simulink model "sim_quadrotor_linear_16b"  (R2016b)
settings: Solver=ode4  StartTime=0.0  StopTime=25  FixedStep=0.0001  RelTol=1e-3
values from neighbouring files (symbols this model uses):
  Par_mdlQuad = mdl_quadrotor_par()    [sim_quadrotor_linear_init.m]
undefined symbols (not defined in the file or in its folder): Ag_phi_rad, Ag_theta_rad, AgVel_p_radPerScnd, AgVel_q_radPerScnd, Pos_z_mtr, V_u_mtrPerScnd, V_v_mtrPerScnd, V_w_mtrPerScnd
settings Model: Creator=Nu  LastModifiedBy=Nu

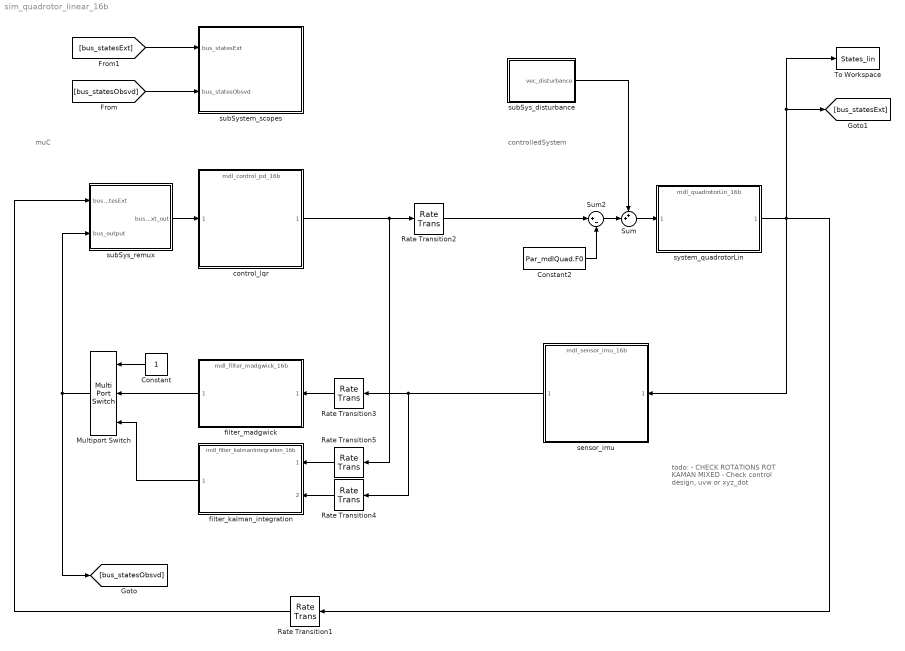
== system sim_quadrotor_linear_16b ==
  note: todo:
      | - CHECK ROTATIONS ROT KAMAN MIXED
      | - Check control design, uvw or xyz_dot
  note: controlledSystem
  note: muC
  Constant : Constant
  Constant2 : Constant  Value=Par_mdlQuad.F0
  Multiport Switch : MultiPortSwitch  DataPortOrder=Zero-based contiguous  Inputs=2
  Rate Transition1 : RateTransition
  Rate Transition2 : RateTransition
  Rate Transition3 : RateTransition  OutPortSampleTime=Par_filterMadgwick.T
  Rate Transition4 : RateTransition  OutPortSampleTime=Par_filterKalman.T
  Rate Transition5 : RateTransition  X0=Par_mdlQuad.PWM0*ones(4,1)
  Sum : Sum  Inputs=++|
  Sum2 : Sum  Inputs=|+-
  To Workspace : ToWorkspace  VariableName=States_lin  SaveFormat=Timeseries  SampleTime=-1
  control_lqr : ModelReference  ModelNameDialog=mdl_control_pd_16b.slx  SimulationMode=Normal  ModelReferenceVersion=1.259
  filter_kalman_integration : ModelReference  ModelNameDialog=mdl_filter_kalmanIntegration_16b.slx  SimulationMode=Normal  ModelReferenceVersion=1.142
  filter_madgwick : ModelReference  ModelNameDialog=mdl_filter_madgwick_16b.slx  SimulationMode=Normal  ModelReferenceVersion=1.85
  sensor_imu : ModelReference  ModelNameDialog=mdl_sensor_imu_16b.slx  SimulationMode=Normal  ModelReferenceVersion=1.279
  subSys_disturbance : Subsystem
  subSys_remux : Subsystem
  subSystem_scopes : Subsystem
  system_quadrotorLin : ModelReference  ModelNameDialog=mdl_quadrotorLin_16b.slx  SimulationMode=Normal  ModelReferenceVersion=1.303
  wires:
  system_quadrotorLin/1 -> To Workspace/1, [bus_statesExt], Rate Transition1/1, sensor_imu/1
  sensor_imu/1 -> Rate Transition4/1, Rate Transition3/1
  [bus_statesObsvd] -> subSystem_scopes/2(bus_statesObsvd)
  [bus_statesExt] -> subSystem_scopes/1(bus_statesExt)
  Multiport Switch/1 -> [bus_statesObsvd], subSys_remux/2(bus_output)
  Rate Transition3/1 -> filter_madgwick/1
  filter_kalman_integration/1 -> Multiport Switch/3
  filter_madgwick/1 -> Multiport Switch/2
  Constant/1 -> Multiport Switch/1
  Rate Transition4/1 -> filter_kalman_integration/2
  Rate Transition1/1 -> subSys_remux/1(bus_statesExt)
  subSys_remux/1(bus_statesExt_out) -> control_lqr/1
  Rate Transition5/1 -> filter_kalman_integration/1
  control_lqr/1 -> Rate Transition2/1, Rate Transition5/1
  subSys_disturbance/1(vec_disturbance) -> Sum/1
  Rate Transition2/1 -> Sum2/1
  Constant2/1 -> Sum2/2
  Sum2/1 -> Sum/2
  Sum/1 -> system_quadrotorLin/1

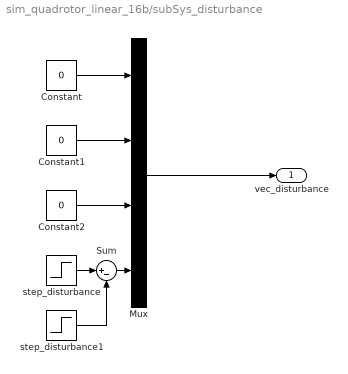
== system sim_quadrotor_linear_16b/subSys_disturbance ==
  Constant : Constant  Value=0
  Constant1 : Constant  Value=0
  Constant2 : Constant  Value=0
  Mux : Mux
  Sum : Sum  Inputs=|+-
  step_disturbance : Step  Time=10  After=0.1  SampleTime=0
  step_disturbance1 : Step  Time=10.5  After=0.1  SampleTime=0
  vec_disturbance : Outport
  wires:
  Sum/1 -> Mux/4
  Constant/1 -> Mux/1
  Constant1/1 -> Mux/2
  Constant2/1 -> Mux/3
  step_disturbance1/1 -> Sum/2
  step_disturbance/1 -> Sum/1
  Mux/1 -> vec_disturbance/1

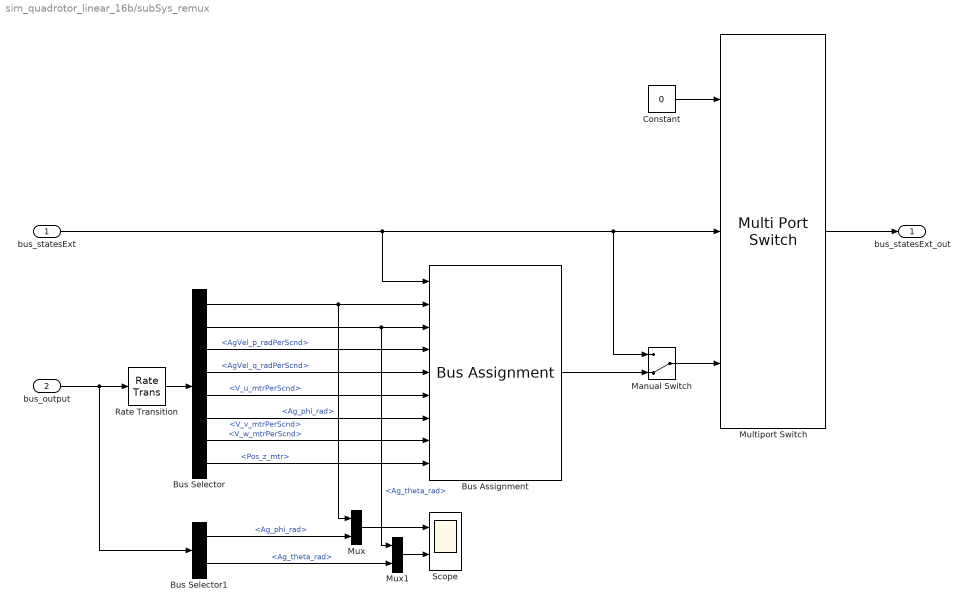
== system sim_quadrotor_linear_16b/subSys_remux ==
  bus_statesExt : Inport
  bus_output : Inport  Port=2
  Bus Assignment : BusAssignment  AssignedSignals=Ag_phi_rad,Ag_theta_rad,AgVel_p_radPerScnd,AgVel_q_radPerScnd,V_u_mtrPerScnd,V_v_mtrPerScnd,V_w_mtrPerScnd,Pos_z_mtr
  Bus Selector : BusSelector  OutputSignals=Ag_phi_rad,Ag_theta_rad,AgVel_p_radPerScnd,AgVel_q_radPerScnd,V_u_mtrPerScnd,V_v_mtrPerScnd,V_w_mtrPerScnd,Pos_z_mtr
  Bus Selector1 : BusSelector  OutputSignals=Ag_phi_rad,Ag_theta_rad
  Constant : Constant  Value=0
  Manual Switch : ManualSwitch  CurrentSetting=0
  Multiport Switch : MultiPortSwitch  DataPortOrder=Zero-based contiguous  Inputs=2
  Mux : Mux  Inputs=2
  Mux1 : Mux  Inputs=2
  Rate Transition : RateTransition
  Scope : Scope  NumInputPorts=2
  bus_statesExt_out : Outport
  wires:
  Bus Selector/2 -> Mux1/1, Bus Assignment/3  "<Ag_theta_rad>"
  Bus Selector/1 -> Mux/1, Bus Assignment/2  "<Ag_phi_rad>"
  Multiport Switch/1 -> bus_statesExt_out/1
  Constant/1 -> Multiport Switch/1
  bus_statesExt/1 -> Manual Switch/1, Multiport Switch/2, Bus Assignment/1
  bus_output/1 -> Rate Transition/1, Bus Selector1/1
  Bus Assignment/1 -> Manual Switch/2
  Rate Transition/1 -> Bus Selector/1
  Bus Selector1/1 -> Mux/2  "<Ag_phi_rad>"
  Mux/1 -> Scope/1
  Mux1/1 -> Scope/2
  Bus Selector1/2 -> Mux1/2  "<Ag_theta_rad>"
  Bus Selector/3 -> Bus Assignment/4  "<AgVel_p_radPerScnd>"
  Bus Selector/4 -> Bus Assignment/5  "<AgVel_q_radPerScnd>"
  Bus Selector/5 -> Bus Assignment/6  "<V_u_mtrPerScnd>"
  Bus Selector/6 -> Bus Assignment/7  "<V_v_mtrPerScnd>"
  Manual Switch/1 -> Multiport Switch/3
  Bus Selector/7 -> Bus Assignment/8  "<V_w_mtrPerScnd>"
  Bus Selector/8 -> Bus Assignment/9  "<Pos_z_mtr>"

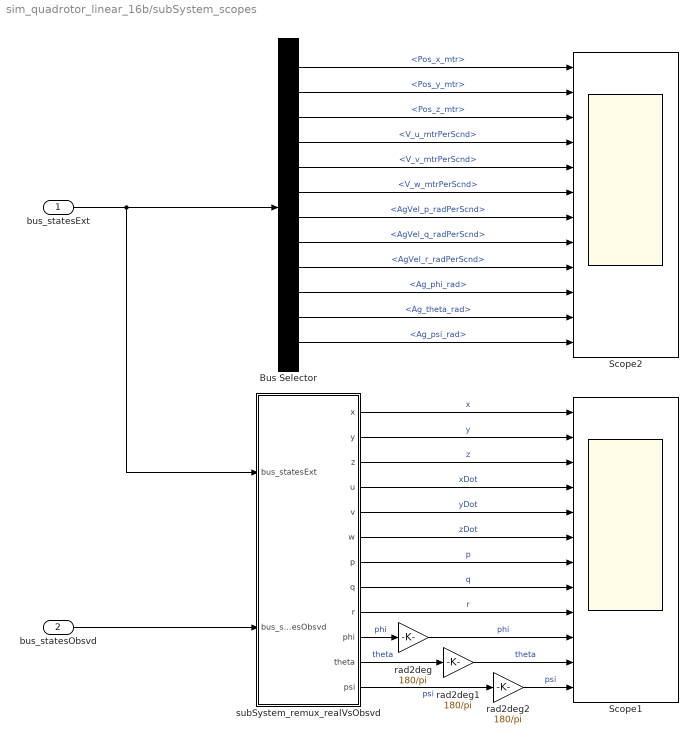
== system sim_quadrotor_linear_16b/subSystem_scopes ==
  bus_statesExt : Inport
  bus_statesObsvd : Inport  Port=2
  Bus Selector : BusSelector  OutputSignals=Pos_x_mtr,Pos_y_mtr,Pos_z_mtr,V_u_mtrPerScnd,V_v_mtrPerScnd,V_w_mtrPerScnd,AgVel_p_radPerScnd,AgVel_q_radPerScnd,AgVel_r_radPerScnd,Ag_phi_rad,Ag_theta_rad,Ag_psi_rad
  Scope1 : Scope  NumInputPorts=12
  Scope2 : Scope  NumInputPorts=12
  rad2deg : Gain  Gain=180/pi
  rad2deg1 : Gain  Gain=180/pi
  rad2deg2 : Gain  Gain=180/pi
  subSystem_remux_realVsObsvd : Subsystem
  wires:
  subSystem_remux_realVsObsvd/1(x) -> Scope1/1  "x"
  subSystem_remux_realVsObsvd/2(y) -> Scope1/2  "y"
  subSystem_remux_realVsObsvd/3(z) -> Scope1/3  "z"
  subSystem_remux_realVsObsvd/7(p) -> Scope1/7  "p"
  subSystem_remux_realVsObsvd/8(q) -> Scope1/8  "q"
  subSystem_remux_realVsObsvd/9(r) -> Scope1/9  "r"
  subSystem_remux_realVsObsvd/10(phi) -> rad2deg/1  "phi"
  subSystem_remux_realVsObsvd/11(theta) -> rad2deg1/1  "theta"
  subSystem_remux_realVsObsvd/12(psi) -> rad2deg2/1  "psi"
  bus_statesExt/1 -> Bus Selector/1, subSystem_remux_realVsObsvd/1(bus_statesExt)
  bus_statesObsvd/1 -> subSystem_remux_realVsObsvd/2(bus_statesObsvd)
  rad2deg/1 -> Scope1/10  "phi"
  rad2deg1/1 -> Scope1/11  "theta"
  rad2deg2/1 -> Scope1/12  "psi"
  Bus Selector/1 -> Scope2/1  "<Pos_x_mtr>"
  Bus Selector/2 -> Scope2/2  "<Pos_y_mtr>"
  Bus Selector/3 -> Scope2/3  "<Pos_z_mtr>"
  Bus Selector/4 -> Scope2/4  "<V_u_mtrPerScnd>"
  Bus Selector/5 -> Scope2/5  "<V_v_mtrPerScnd>"
  Bus Selector/6 -> Scope2/6  "<V_w_mtrPerScnd>"
  Bus Selector/7 -> Scope2/7  "<AgVel_p_radPerScnd>"
  Bus Selector/8 -> Scope2/8  "<AgVel_q_radPerScnd>"
  Bus Selector/9 -> Scope2/9  "<AgVel_r_radPerScnd>"
  Bus Selector/10 -> Scope2/10  "<Ag_phi_rad>"
  Bus Selector/11 -> Scope2/11  "<Ag_theta_rad>"
  Bus Selector/12 -> Scope2/12  "<Ag_psi_rad>"
  subSystem_remux_realVsObsvd/4(u) -> Scope1/4  "xDot"
  subSystem_remux_realVsObsvd/5(v) -> Scope1/5  "yDot"
  subSystem_remux_realVsObsvd/6(w) -> Scope1/6  "zDot"

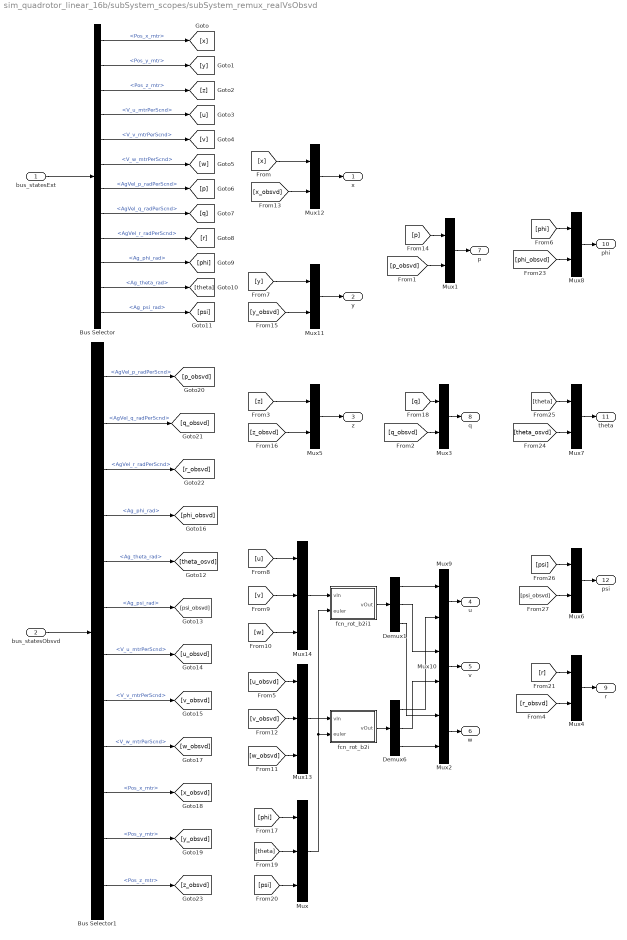
== system sim_quadrotor_linear_16b/subSystem_scopes/subSystem_remux_realVsObsvd ==
  bus_statesExt : Inport
  bus_statesObsvd : Inport  Port=2
  Bus Selector : BusSelector  OutputSignals=Pos_x_mtr,Pos_y_mtr,Pos_z_mtr,V_u_mtrPerScnd,V_v_mtrPerScnd,V_w_mtrPerScnd,AgVel_p_radPerScnd,AgVel_q_radPerScnd,AgVel_r_radPerScnd,Ag_phi_rad,Ag_theta_rad,Ag_psi_rad
  Bus Selector1 : BusSelector  OutputSignals=AgVel_p_radPerScnd,AgVel_q_radPerScnd,AgVel_r_radPerScnd,Ag_phi_rad,Ag_theta_rad,Ag_psi_rad,V_u_mtrPerScnd,V_v_mtrPerScnd,V_w_mtrPerScnd,Pos_x_mtr,Pos_y_mtr,Pos_z_mtr
  Demux1 : Demux  Outputs=3
  Demux6 : Demux  Outputs=3
  Mux : Mux  Inputs=3
  Mux{1..12} (12 alike) : Mux  Inputs=2
  Mux13 : Mux  Inputs=3
  Mux14 : Mux  Inputs=3
  fcn_rot_b2i : MATLAB Function  TreatAsAtomicUnit=on
  fcn_rot_b2i1 : MATLAB Function  TreatAsAtomicUnit=on
  x : Outport
  y : Outport  Port=2
  z : Outport  Port=3
  u : Outport  Port=4
  v : Outport  Port=5
  w : Outport  Port=6
  p : Outport  Port=7
  q : Outport  Port=8
  r : Outport  Port=9
  phi : Outport  Port=10
  theta : Outport  Port=11
  psi : Outport  Port=12
  wires:
  [z] -> Mux5/1
  [z_obsvd] -> Mux5/2
  Bus Selector1/3 -> [r_obsvd]  "<AgVel_r_radPerScnd>"
  Bus Selector1/2 -> [q_obsvd]  "<AgVel_q_radPerScnd>"
  Bus Selector1/1 -> [p_obsvd]  "<AgVel_p_radPerScnd>"
  Bus Selector/9 -> [r]  "<AgVel_r_radPerScnd>"
  Bus Selector/10 -> [phi]  "<Ag_phi_rad>"
  Bus Selector/11 -> [theta]  "<Ag_theta_rad>"
  Bus Selector/12 -> [psi]  "<Ag_psi_rad>"
  Bus Selector/8 -> [q]  "<AgVel_q_radPerScnd>"
  Bus Selector/7 -> [p]  "<AgVel_p_radPerScnd>"
  Bus Selector/6 -> [w]  "<V_w_mtrPerScnd>"
  Bus Selector/5 -> [v]  "<V_v_mtrPerScnd>"
  Bus Selector/4 -> [u]  "<V_u_mtrPerScnd>"
  Bus Selector/2 -> [y]  "<Pos_y_mtr>"
  Bus Selector/3 -> [z]  "<Pos_z_mtr>"
  Mux2/1 -> w/1
  Mux5/1 -> z/1
  bus_statesObsvd/1 -> Bus Selector1/1
  bus_statesExt/1 -> Bus Selector/1
  Bus Selector/1 -> [x]  "<Pos_x_mtr>"
  [w] -> Mux14/3
  [w_obsvd] -> Mux13/3
  [p] -> Mux1/1
  [p_obsvd] -> Mux1/2
  [q] -> Mux3/1
  [q_obsvd] -> Mux3/2
  [r] -> Mux4/1
  [r_obsvd] -> Mux4/2
  [psi] -> Mux6/1
  [psi_obsvd] -> Mux6/2
  [theta] -> Mux7/1
  [theta_osvd] -> Mux7/2
  [phi] -> Mux8/1
  [phi_obsvd] -> Mux8/2
  Mux1/1 -> p/1
  Mux3/1 -> q/1
  Mux4/1 -> r/1
  Mux6/1 -> psi/1
  Mux7/1 -> theta/1
  Mux8/1 -> phi/1
  Bus Selector1/5 -> [theta_osvd]  "<Ag_theta_rad>"
  Bus Selector1/6 -> [psi_obsvd]  "<Ag_psi_rad>"
  Bus Selector1/4 -> [phi_obsvd]  "<Ag_phi_rad>"
  Bus Selector1/7 -> [u_obsvd]  "<V_u_mtrPerScnd>"
  Bus Selector1/8 -> [v_obsvd]  "<V_v_mtrPerScnd>"
  Bus Selector1/9 -> [w_obsvd]  "<V_w_mtrPerScnd>"
  Mux9/1 -> u/1
  [u] -> Mux14/1
  [u_obsvd] -> Mux13/1
  Mux10/1 -> v/1
  [v] -> Mux14/2
  [v_obsvd] -> Mux13/2
  Bus Selector1/12 -> [z_obsvd]  "<Pos_z_mtr>"
  Bus Selector1/11 -> [y_obsvd]  "<Pos_y_mtr>"
  Bus Selector1/10 -> [x_obsvd]  "<Pos_x_mtr>"
  [y_obsvd] -> Mux11/2
  [y] -> Mux11/1
  Mux11/1 -> y/1
  [x_obsvd] -> Mux12/2
  [x] -> Mux12/1
  Mux12/1 -> x/1
  Mux13/1 -> fcn_rot_b2i/1(vIn)
  fcn_rot_b2i/1(vOut) -> Demux6/1
  Mux14/1 -> fcn_rot_b2i1/1(vIn)
  fcn_rot_b2i1/1(vOut) -> Demux1/1
  Demux1/1 -> Mux9/1
  Demux6/1 -> Mux9/2
  Demux1/2 -> Mux10/1
  Demux6/2 -> Mux10/2
  Demux1/3 -> Mux2/1
  Demux6/3 -> Mux2/2
  [phi] -> Mux/1
  [theta] -> Mux/2
  [psi] -> Mux/3
  Mux/1 -> fcn_rot_b2i/2(euler), fcn_rot_b2i1/2(euler)

== matlab function sim_quadrotor_linear_16b/subSystem_scopes/subSystem_remux_realVsObsvd/fcn_rot_b2i ==
  data: vIn input; euler input; vOut output
function vOut = fcn(vIn, euler)

vOut    = rot_euler(vIn, euler, 'to-inertial-frame');

== matlab function sim_quadrotor_linear_16b/subSystem_scopes/subSystem_remux_realVsObsvd/fcn_rot_b2i1 ==
  data: vIn input; euler input; vOut output
function vOut = fcn(vIn, euler)

vOut    = rot_euler(vIn, euler, 'to-inertial-frame');
